simulink model "ex3S"  (R2022a)
settings: Solver=VariableStepAuto  StartTime=0.0  StopTime=10.0  RelTol=1e-3
settings Model: Creator=giova  LastModifiedBy=giova

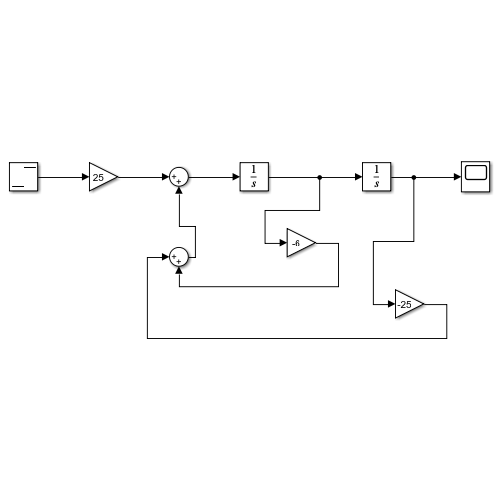
[thumbnail: Simulink's stored preview of the top-level diagram]
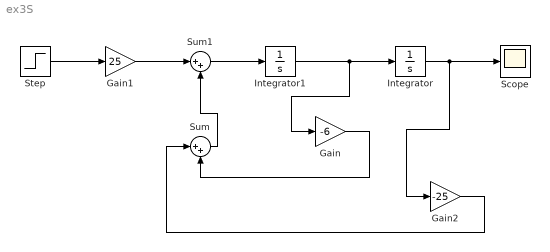
== system ex3S ==
  Gain : Gain  Gain=-6
  Gain1 : Gain  Gain=25
  Gain2 : Gain  Gain=-25
  Integrator : Integrator
  Integrator1 : Integrator
  Scope : Scope
  Step : Step  SampleTime=0
  Sum : Sum  Inputs=|++
  Sum1 : Sum  Inputs=|++
  wires:
  Sum1/1 -> Integrator1/1
  Sum/1 -> Sum1/2
  Integrator/1 -> Scope/1, Gain2/1
  Integrator1/1 -> Gain/1, Integrator/1
  Gain/1 -> Sum/2
  Gain2/1 -> Sum/1
  Gain1/1 -> Sum1/1
  Step/1 -> Gain1/1
